simulink model "exampleTemperature_Conductivity"  (Simulink 8.8)
settings: Solver=VariableStepAuto  StartTime=0.0  StopTime=10.0  RelTol=1e-3  EnableMultiTasking=on
libraries: carnot x4
settings Model: Creator=drhf  LastModifiedBy=drhf
settings OptimizationCC: ExpressionDepthLimit=2147483647
settings DebuggingCC: SolverPrmCheckMsg=warning

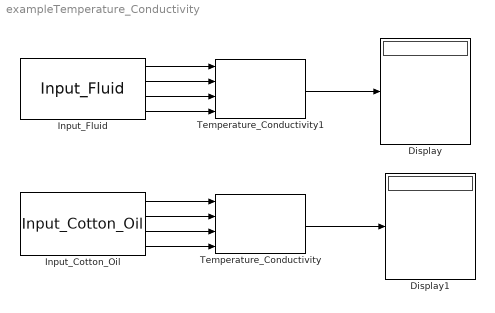
== system exampleTemperature_Conductivity ==
  Display : Display
  Display1 : Display
  Input_Cotton_Oil : carnot/Basic/Material_Properties/Input_Cotton_Oil  T=[10:10:50]  p=1e5
  Input_Fluid : carnot/Basic/Material_Properties/Input_Fluid  fluid=Water  T=[10:10:50]  p=1e5  x=0.005
  Temperature_Conductivity : carnot/Basic/Material_Properties/Temperature_Conductivity  VariantControl=CarlibClassic  INPUTARGUMENTS=state variables (classic)  DEBUGLEVEL=WARNINGLEVEL  MAXTOTALMESSAGES=inf  MAXCONSECUTIVEMESSAGES=inf  WRITETOFILE=0  FILENAME='errors.txt'
  Temperature_Conductivity1 : carnot/Basic/Material_Properties/Temperature_Conductivity  VariantControl=CarlibClassic  INPUTARGUMENTS=state variables (classic)  DEBUGLEVEL=WARNINGLEVEL  MAXTOTALMESSAGES=inf  MAXCONSECUTIVEMESSAGES=inf  WRITETOFILE=0  FILENAME='errors.txt'
  wires:
  Input_Fluid/1 -> Temperature_Conductivity1/1
  Input_Fluid/2 -> Temperature_Conductivity1/2
  Input_Fluid/3 -> Temperature_Conductivity1/3
  Input_Fluid/4 -> Temperature_Conductivity1/4
  Temperature_Conductivity1/1 -> Display/1
  Input_Cotton_Oil/1 -> Temperature_Conductivity/1
  Input_Cotton_Oil/2 -> Temperature_Conductivity/2
  Input_Cotton_Oil/3 -> Temperature_Conductivity/3
  Input_Cotton_Oil/4 -> Temperature_Conductivity/4
  Temperature_Conductivity/1 -> Display1/1
